simulink model "atrias_HW_boom_nmSt_kinSw_v4"  (R2015a)
settings: Solver=ode4  StartTime=0.0  StopTime=inf  FixedStep=sample_time  RelTol=1e-3
values from neighbouring files (symbols this model uses):
  control_start_time = 15    [setParams.m]
  flag_CtrlMode = 0    [setParams.m]
  kinSw_alpha_start = 130*pi/180    (= 2.26892802759)    [setParams.m]
  kinSw_alpha_tgt = 70*pi/180    (= 1.2217304764)    [setParams.m]
  kinSw_t_start = 0.5    [setParams.m]
  poser_LLegAlp = (initial_l_leg_angle -pi/2)*180/pi    (= 105)    [setParams.m]
  poser_LLegLen = initial_l_leg_length    (= 0.8)    [setParams.m]
  poser_RLegAlp = (initial_r_leg_angle -pi/2)*180/pi    (= 75)    [setParams.m]
  poser_RLegLen = initial_r_leg_length    (= 0.8)    [setParams.m]
  tune_kinSw_alpha_start = kinSw_alpha_start*180/pi    (= 130)    [setParams.m]
  tune_kinSw_alpha_tgt = kinSw_alpha_tgt*180/pi    (= 70)    [setParams.m]
  tune_kinSw_gClr_tgt = kinSw_gClr    (= 0.15)    [setParams.m]
  tune_kinSw_gH_tgt = kinSw_gH_tgt    (= -0.01)    [setParams.m]
  tune_M1_G = 9.5    [setParams.m]
  tune_M3_0 = CtrlPar_theta0*180/pi    [setParams.m]
  tune_M3_D = St_GainDTh_HFL*5    [setParams.m]
  tune_M3_P = St_GainTh_HFL*5    [setParams.m]
  tune_M4_G = 1    [setParams.m]
undefined symbols (not defined in the file or in its folder): A1_notch_f1, A2_notch_f1, A_kalman_fourbar_gear, A_lpf_dtau, B1_lpf_dtau, B1_notch_f1, B2_lpf_dtau, B2_notch_f1, B_kalman_fourbar_gear, boom_mount_angle, boom_mount_to_center_diagonal, c_jointstop, C_kalman_fourbar_gear, contactThr, d_vertical_com, delta_phi_max, delta_phi_max_buffer, delta_phi_max_dropoff, delta_phi_min, Discrete, FmaxBFSH, FmaxGLU, FmaxHAM, FmaxHFL, FmaxRF, FmaxVAS, FPCtrlPar, g, gain_nodes_sea_torque, HIP_MTR_MAX_CONT_TORQUE, initial_dx_estimate, j_motor, k_leg_spring, K_notch_f1, k_sea, kalman_load_to_deflect_transmission, kd_lateral, kd_motor, kd_shin_max, kd_shin_min, kd_splay_max, kd_splay_min, kd_thigh_max, kd_thigh_min, kp_lateral, kp_motor, kp_sea_torque, kp_shin_max, kp_shin_min, kp_splay_max, kp_splay_min, kp_thigh_max, kp_thigh_min, l_boom, l_seg, l_v, lateral_motor_efficiency, lateral_offset, lateral_target_angle_right, lateral_transition_force ... (+123)
libraries: simulink_extras x28, simulink x11, ctrlSharedLib x4
(part 5 of 8)

== system atrias_HW_boom_nmSt_kinSw_v4/Control/Behavior Control/Virtual Neuromuscular Control/Neural Control Layer/L Stance Phase (sagittal) ==
  note: Left Stance Phase Control
  note: 0: Prestimulations
  note: M1: realize compliant leg
  note: M2: prevent knee overextension
  note: M3: balance trunk
  CtrlPar : Inport
  theta_tgt [rad] : Inport  Port=2
  theta dtheta [rad rad/s] : Inport  Port=3
  FmVAS : Inport  Port=4
  LceBFSH : Inport  Port=5
  Enable : EnablePort  StatesWhenEnabling=reset  ZeroCross=off
  Demux2 : Demux
  Demux5 : Demux  Outputs=5
  Demux7 : Demux  Outputs=2
  Divide{4..6,8,13,15,19..20} (8 alike) : Product
  Gain : Gain  Gain=-1
  Gain2 : Gain  Gain=-1
  Gain3 : Gain  Gain=-1
  Mux1 : Mux  Inputs=3
  Mux2 : Mux  Inputs=2
  Sum1 : Sum  Inputs=-+|  SaturateOnIntegerOverflow=on  InputSameDT=on  OutDataTypeStr=Inherit: Same as first input
  Sum2 : Sum  Inputs=|++  SaturateOnIntegerOverflow=on  InputSameDT=on  OutDataTypeStr=Inherit: Same as first input
  Sum3 : Sum  Inputs=-+|  SaturateOnIntegerOverflow=on  InputSameDT=on  OutDataTypeStr=Inherit: Same as first input
  Sum4 : Sum  Inputs=-+|  SaturateOnIntegerOverflow=on  InputSameDT=on  OutDataTypeStr=Inherit: Same as first input
  Sum8 : Sum  Inputs=|++  SaturateOnIntegerOverflow=on  InputSameDT=on  OutDataTypeStr=Inherit: Same as first input
  parStPreS : Selector  InputPortWidth=St_i  Indices=parSt_PreS_i
  parSt_M1 : Selector  InputPortWidth=St_i  Indices=parSt_M1_i
  parSt_M2 : Selector  InputPortWidth=St_i  Indices=parSt_M2_i
  parSt_M3 : Selector  InputPortWidth=St_i  Indices=parSt_M3_i
  positive half{1..4,6} (5 alike) : Saturate  UpperLimit=inf  LowerLimit=0  ZeroCross=off
  S_St_0 : Outport  OutputWhenDisabled=reset  InitialOutput=0
  S_M1 [VAS] : Outport  Port=2  OutputWhenDisabled=reset  InitialOutput=0
  S_M2 [VAS BFSH] : Outport  Port=3  OutputWhenDisabled=reset  InitialOutput=0
  S_M3 [HFL GLU HAM] : Outport  Port=4  OutputWhenDisabled=reset  InitialOutput=0
  wires:
  CtrlPar/1 -> parStPreS/1, parSt_M3/1, parSt_M2/1, parSt_M1/1
  parStPreS/1 -> S_St_0/1
  parSt_M1/1 -> Divide8/1  "FGain_VAS"
  Divide8/1 -> S_M1 [VAS]/1  "VAS"
  FmVAS/1 -> Divide8/2
  parSt_M2/1 -> Demux2/1
  Sum3/1 -> positive half3/1
  Demux2/2 -> Divide15/2  "LGainBFSH_VAS"
  Demux2/4 -> Divide13/2  "LGain_BFSH"
  positive half3/1 -> Divide15/1
  Demux2/1 -> Sum3/1  "loff_BFSH_VAS"
  Divide15/1 -> Gain/1
  Divide13/1 -> Mux2/2  "BFSH"
  Gain/1 -> Mux2/1  "VAS"
  Sum4/1 -> positive half4/1
  positive half4/1 -> Divide13/1
  Demux2/3 -> Sum4/1  "loff_BFSH"
  LceBFSH/1 -> Sum3/2, Sum4/2
  Mux2/1 -> S_M2 [VAS BFSH]/1
  parSt_M3/1 -> Demux5/1
  Demux5/1 -> Divide19/2  "GainTh_HFL"
  Demux5/2 -> Divide20/2  "GainDTh_HFL"
  Demux5/3 -> Divide4/2  "GainTh_GLU"
  Demux5/4 -> Divide5/2  "GainDTh_GLU"
  theta dtheta [rad rad/s]/1 -> Demux7/1
  Demux7/1 -> Sum1/2  "theta"
  Demux7/2 -> Gain3/1, Divide5/1  "dtheta"
  Sum1/1 -> Gain2/1, Divide4/1
  Gain2/1 -> Divide19/1
  Gain3/1 -> Divide20/1
  Divide19/1 -> Sum2/1
  Divide20/1 -> Sum2/2
  Divide4/1 -> Sum8/1
  Divide5/1 -> Sum8/2
  Sum2/1 -> positive half1/1  "HFL"
  Sum8/1 -> Divide6/1, positive half2/1  "GLU"
  Mux1/1 -> S_M3 [HFL GLU HAM]/1
  Demux5/5 -> Divide6/2  "SGainGLU_HAM"
  Divide6/1 -> positive half6/1  "HAM"
  theta_tgt [rad]/1 -> Sum1/1
  positive half1/1 -> Mux1/1
  positive half2/1 -> Mux1/2
  positive half6/1 -> Mux1/3

== system atrias_HW_boom_nmSt_kinSw_v4/Control/Behavior Control/Virtual Neuromuscular Control/Neural Control Layer/L Stance, Swing, Trans (sagittal) ==
  note: Stance DS1 Swing DS2
  note: FullStance Swing
  note: |------------------------------|--------------------|
  note: |--------------------|------------------------------|
  ILLoad : Inport
  S_0_St : Inport  Port=2
  S_M1 : Inport  Port=3
  S_M2 : Inport  Port=4
  S_M3 : Inport  Port=5
  Add3 : Sum  Inputs=2
  Demux2 : Demux  Outputs=2
  Demux3 : Demux  Outputs=3
  Divide17 : Product
  Mux1 : Mux  Inputs=7
  Mux6 : Mux  Inputs=6
  RF : Constant  Value=0
  Sum6 : Sum  Inputs=++|  SaturateOnIntegerOverflow=on  InputSameDT=on  OutDataTypeStr=Inherit: Same as first input
  S : Outport  OutputWhenDisabled=reset  InitialOutput=0
  S_Modules : Outport  Port=2  OutputWhenDisabled=reset  InitialOutput=0
  wires:
  [M3_HFL] -> Mux6/1  "HFL"
  [M3_GLU] -> Mux6/2  "GLU"
  [M3_HAM] -> Mux6/3  "HAM"
  Add3/1 -> Mux6/5  "VAS"
  [M2_BFSH] -> Mux6/6  "KFL"
  Mux6/1 -> Sum6/2
  Sum6/1 -> S/1
  S_0_St/1 -> Sum6/1, [M0_St]
  S_M1/1 -> [M1_VAS]  "VAS"
  S_M2/1 -> Demux2/1  "VAS BFSH"
  Demux2/1 -> [M2_VAS]  "M2_VAS"
  Demux2/2 -> [M2_BFSH]  "M2_BFSH"
  S_M3/1 -> Divide17/1
  ILLoad/1 -> Divide17/2
  Divide17/1 -> Demux3/1
  Demux3/1 -> [M3_HFL]  "M3_HFL"
  Demux3/2 -> [M3_GLU]  "M3_GLU"
  Demux3/3 -> [M3_HAM]  "M3_HAM"
  [M1_VAS] -> Add3/1
  [M2_VAS] -> Add3/2
  [M3_HFL] -> Mux1/5  "10"
  [M3_GLU] -> Mux1/6  "11"
  [M3_HAM] -> Mux1/7  "12"
  [M2_VAS] -> Mux1/3  "8"
  [M2_BFSH] -> Mux1/4  "9"
  [M1_VAS] -> Mux1/2  "7"
  [M0_St] -> Mux1/1  "1~6"
  Mux1/1 -> S_Modules/1
  RF/1 -> Mux6/4

== system atrias_HW_boom_nmSt_kinSw_v4/Control/Behavior Control/Virtual Neuromuscular Control/Neural Control Layer/R Stance Phase (sagittal) ==
  note: Left Stance Phase Control
  note: 0: Prestimulations
  note: M1: realize compliant leg
  note: M2: prevent knee overextension
  note: M3: balance trunk
  CtrlPar : Inport
  theta_tgt [rad] : Inport  Port=2
  theta dtheta [rad rad/s] : Inport  Port=3
  FmVAS : Inport  Port=4
  LceBFSH : Inport  Port=5
  Enable : EnablePort  StatesWhenEnabling=reset  ZeroCross=off
  Demux2 : Demux
  Demux5 : Demux  Outputs=5
  Demux7 : Demux  Outputs=2
  Divide{4..6,8,13,15,19..20} (8 alike) : Product
  Gain : Gain  Gain=-1
  Gain2 : Gain  Gain=-1
  Gain3 : Gain  Gain=-1
  Mux1 : Mux  Inputs=3
  Mux2 : Mux  Inputs=2
  Sum1 : Sum  Inputs=-+|  SaturateOnIntegerOverflow=on  InputSameDT=on  OutDataTypeStr=Inherit: Same as first input
  Sum2 : Sum  Inputs=|++  SaturateOnIntegerOverflow=on  InputSameDT=on  OutDataTypeStr=Inherit: Same as first input
  Sum3 : Sum  Inputs=-+|  SaturateOnIntegerOverflow=on  InputSameDT=on  OutDataTypeStr=Inherit: Same as first input
  Sum4 : Sum  Inputs=-+|  SaturateOnIntegerOverflow=on  InputSameDT=on  OutDataTypeStr=Inherit: Same as first input
  Sum8 : Sum  Inputs=|++  SaturateOnIntegerOverflow=on  InputSameDT=on  OutDataTypeStr=Inherit: Same as first input
  parStPreS : Selector  InputPortWidth=St_i  Indices=parSt_PreS_i
  parSt_M1 : Selector  InputPortWidth=St_i  Indices=parSt_M1_i
  parSt_M2 : Selector  InputPortWidth=St_i  Indices=parSt_M2_i
  parSt_M3 : Selector  InputPortWidth=St_i  Indices=parSt_M3_i
  positive half{1..4,6} (5 alike) : Saturate  UpperLimit=inf  LowerLimit=0  ZeroCross=off
  S_St_0 : Outport  OutputWhenDisabled=reset  InitialOutput=0
  S_M1 [VAS] : Outport  Port=2  OutputWhenDisabled=reset  InitialOutput=0
  S_M2 [VAS BFSH] : Outport  Port=3  OutputWhenDisabled=reset  InitialOutput=0
  S_M3 [HFL GLU HAM] : Outport  Port=4  OutputWhenDisabled=reset  InitialOutput=0
  wires:
  CtrlPar/1 -> parStPreS/1, parSt_M3/1, parSt_M2/1, parSt_M1/1
  parStPreS/1 -> S_St_0/1
  parSt_M1/1 -> Divide8/1  "FGain_VAS"
  Divide8/1 -> S_M1 [VAS]/1  "VAS"
  FmVAS/1 -> Divide8/2
  parSt_M2/1 -> Demux2/1
  Sum3/1 -> positive half3/1
  Demux2/2 -> Divide15/2  "LGainBFSH_VAS"
  Demux2/4 -> Divide13/2  "LGain_BFSH"
  positive half3/1 -> Divide15/1
  Demux2/1 -> Sum3/1  "loff_BFSH_VAS"
  Divide15/1 -> Gain/1
  Divide13/1 -> Mux2/2  "BFSH"
  Gain/1 -> Mux2/1  "VAS"
  Sum4/1 -> positive half4/1
  positive half4/1 -> Divide13/1
  Demux2/3 -> Sum4/1  "loff_BFSH"
  LceBFSH/1 -> Sum3/2, Sum4/2
  Mux2/1 -> S_M2 [VAS BFSH]/1
  parSt_M3/1 -> Demux5/1
  Demux5/1 -> Divide19/2  "GainTh_HFL"
  Demux5/2 -> Divide20/2  "GainDTh_HFL"
  Demux5/3 -> Divide4/2  "GainTh_GLU"
  Demux5/4 -> Divide5/2  "GainDTh_GLU"
  theta dtheta [rad rad/s]/1 -> Demux7/1
  Demux7/1 -> Sum1/2  "theta"
  Demux7/2 -> Gain3/1, Divide5/1  "dtheta"
  Sum1/1 -> Gain2/1, Divide4/1
  Gain2/1 -> Divide19/1
  Gain3/1 -> Divide20/1
  Divide19/1 -> Sum2/1
  Divide20/1 -> Sum2/2
  Divide4/1 -> Sum8/1
  Divide5/1 -> Sum8/2
  Sum2/1 -> positive half1/1  "HFL"
  Sum8/1 -> Divide6/1, positive half2/1  "GLU"
  Mux1/1 -> S_M3 [HFL GLU HAM]/1
  Demux5/5 -> Divide6/2  "SGainGLU_HAM"
  Divide6/1 -> positive half6/1  "HAM"
  theta_tgt [rad]/1 -> Sum1/1
  positive half1/1 -> Mux1/1
  positive half2/1 -> Mux1/2
  positive half6/1 -> Mux1/3

== system atrias_HW_boom_nmSt_kinSw_v4/Control/Behavior Control/Virtual Neuromuscular Control/Neural Control Layer/R Stance, Swing, Trans (sagittal) ==
  note: Stance DS1 Swing DS2
  note: FullStance Swing
  note: |------------------------------|--------------------|
  note: |--------------------|------------------------------|
  ILLoad : Inport
  S_0_St : Inport  Port=2
  S_M1 : Inport  Port=3
  S_M2 : Inport  Port=4
  S_M3 : Inport  Port=5
  Add3 : Sum  Inputs=2
  Demux2 : Demux  Outputs=2
  Demux3 : Demux  Outputs=3
  Divide17 : Product
  Mux1 : Mux  Inputs=7
  Mux6 : Mux  Inputs=6
  RF : Constant  Value=0
  Sum6 : Sum  Inputs=++|  SaturateOnIntegerOverflow=on  InputSameDT=on  OutDataTypeStr=Inherit: Same as first input
  S : Outport  OutputWhenDisabled=reset  InitialOutput=0
  S_Modules : Outport  Port=2  OutputWhenDisabled=reset  InitialOutput=0
  wires:
  [M3_HFL] -> Mux6/1  "HFL"
  [M3_GLU] -> Mux6/2  "GLU"
  [M3_HAM] -> Mux6/3  "HAM"
  Add3/1 -> Mux6/5  "VAS"
  [M2_BFSH] -> Mux6/6  "KFL"
  Mux6/1 -> Sum6/2
  Sum6/1 -> S/1
  S_0_St/1 -> Sum6/1, [M0_St]
  S_M1/1 -> [M1_VAS]  "VAS"
  S_M2/1 -> Demux2/1  "VAS BFSH"
  Demux2/1 -> [M2_VAS]  "M2_VAS"
  Demux2/2 -> [M2_BFSH]  "M2_BFSH"
  S_M3/1 -> Divide17/1
  ILLoad/1 -> Divide17/2
  Divide17/1 -> Demux3/1
  Demux3/1 -> [M3_HFL]  "M3_HFL"
  Demux3/2 -> [M3_GLU]  "M3_GLU"
  Demux3/3 -> [M3_HAM]  "M3_HAM"
  [M1_VAS] -> Add3/1
  [M2_VAS] -> Add3/2
  [M3_HFL] -> Mux1/5  "10"
  [M3_GLU] -> Mux1/6  "11"
  [M3_HAM] -> Mux1/7  "12"
  [M2_VAS] -> Mux1/3  "8"
  [M2_BFSH] -> Mux1/4  "9"
  [M1_VAS] -> Mux1/2  "7"
  [M0_St] -> Mux1/1  "1~6"
  Mux1/1 -> S_Modules/1
  RF/1 -> Mux6/4

== system atrias_HW_boom_nmSt_kinSw_v4/Control/Behavior Control/Virtual Neuromuscular Control/Torque Distribution/mech limit avoidance1 ==
  tau_des [Nm]x4 : Inport
  PD Joint Limit : Subsystem
  PD Joint Limit1 : Subsystem  Commented=on
  Product : Product
  Sum : Sum  Inputs=++|
  tau_des + pd [Nm]x4 : Outport
  wires:
  Product/1 -> Sum/2
  PD Joint Limit/2(des_trq_scale x4) -> Product/1
  Sum/1 -> tau_des + pd [Nm]x4/1
  PD Joint Limit/1(tau_pd_hip_knee [Nm]x4) -> Sum/1
  tau_des [Nm]x4/1 -> Product/2

== system atrias_HW_boom_nmSt_kinSw_v4/Control/Behavior Control/command routing/(M4) Swing Leg Complensation/Swing Leg Compensation ==
  StTorques : Inport
  SwTorques : Inport  Port=2
  M4_G : Inport  Port=3
  Demux : Demux  Outputs=2
  Demux1 : Demux  Outputs=2
  Divide : Product
  Gain : Gain  Gain=.5
  Mux : Mux  Inputs=2
  Sum : Sum  Inputs=|++
  Sum1 : Sum  Inputs=|++
  Sum2 : Sum  Inputs=|++
  StTorques_comp : Outport
  SwTorques_comp : Outport  Port=2
  wires:
  Demux1/1 -> Sum1/1
  Sum/1 -> Gain/1  "SwLegTorque"
  Demux/1 -> Sum/1
  Demux1/2 -> Sum2/1
  Demux/2 -> Sum/2
  StTorques/1 -> Demux1/1
  Mux/1 -> StTorques_comp/1  "StTorques_comp"
  SwTorques/1 -> Demux/1, SwTorques_comp/1
  Sum2/1 -> Mux/2
  Divide/1 -> Sum1/2, Sum2/2
  Sum1/1 -> Mux/1
  Gain/1 -> Divide/1
  M4_G/1 -> Divide/2

== system atrias_HW_boom_nmSt_kinSw_v4/Control/Behavior Control/kinematic swing leg controller/Back//Front Motor PD/Friction Compensation ==
  Right/Left [1/0] : Inport
  Commanded Velocity [rad/s] [back front] : Inport  Port=2
  Product : Product
  Sign : Signum
  Sum1 : Sum
  Switch : Switch  Criteria=u2 ~= 0
  Switch1 : Switch  Criteria=u2 ~= 0
  coulomb_friction_left : Constant  Value=sea_coulomb_friction(3:4)
  coulomb_friction_right : Constant  Value=sea_coulomb_friction(1:2)
  offset_friction_left : Constant  Value=sea_offset_friction(3:4)
  offset_friction_right : Constant  Value=sea_offset_friction(1:2)
  Friction Compensation [Nm] : Outport
  wires:
  Commanded Velocity [rad/s] [back front]/1 -> Sign/1
  Switch/1 -> Sum1/2
  Sum1/1 -> Friction Compensation [Nm]/1
  Product/1 -> Sum1/1
  Right/Left [1/0]/1 -> Switch1/2, Switch/2
  offset_friction_right/1 -> Switch/1
  offset_friction_left/1 -> Switch/3
  coulomb_friction_right/1 -> Switch1/1
  coulomb_friction_left/1 -> Switch1/3
  Switch1/1 -> Product/2
  Sign/1 -> Product/1

== system atrias_HW_boom_nmSt_kinSw_v4/Control/Poser/Subsystem/Back//Front Motor PD/Friction Compensation ==
  Right/Left [1/0] : Inport
  Commanded Velocity [rad/s] [back front] : Inport  Port=2
  Product : Product
  Sign : Signum
  Sum1 : Sum
  Switch : Switch  Criteria=u2 ~= 0
  Switch1 : Switch  Criteria=u2 ~= 0
  coulomb_friction_left : Constant  Value=sea_coulomb_friction(3:4)
  coulomb_friction_right : Constant  Value=sea_coulomb_friction(1:2)
  offset_friction_left : Constant  Value=sea_offset_friction(3:4)
  offset_friction_right : Constant  Value=sea_offset_friction(1:2)
  Friction Compensation [Nm] : Outport
  wires:
  Commanded Velocity [rad/s] [back front]/1 -> Sign/1
  Switch/1 -> Sum1/2
  Sum1/1 -> Friction Compensation [Nm]/1
  Product/1 -> Sum1/1
  Right/Left [1/0]/1 -> Switch1/2, Switch/2
  offset_friction_right/1 -> Switch/1
  offset_friction_left/1 -> Switch/3
  coulomb_friction_right/1 -> Switch1/1
  coulomb_friction_left/1 -> Switch1/3
  Switch1/1 -> Product/2
  Sign/1 -> Product/1

== system atrias_HW_boom_nmSt_kinSw_v4/Control/Poser/Subsystem/Back//Front Motor PD1/Friction Compensation ==
  Right/Left [1/0] : Inport
  Commanded Velocity [rad/s] [back front] : Inport  Port=2
  Product : Product
  Sign : Signum
  Sum1 : Sum
  Switch : Switch  Criteria=u2 ~= 0
  Switch1 : Switch  Criteria=u2 ~= 0
  coulomb_friction_left : Constant  Value=sea_coulomb_friction(3:4)
  coulomb_friction_right : Constant  Value=sea_coulomb_friction(1:2)
  offset_friction_left : Constant  Value=sea_offset_friction(3:4)
  offset_friction_right : Constant  Value=sea_offset_friction(1:2)
  Friction Compensation [Nm] : Outport
  wires:
  Commanded Velocity [rad/s] [back front]/1 -> Sign/1
  Switch/1 -> Sum1/2
  Sum1/1 -> Friction Compensation [Nm]/1
  Product/1 -> Sum1/1
  Right/Left [1/0]/1 -> Switch1/2, Switch/2
  offset_friction_right/1 -> Switch/1
  offset_friction_left/1 -> Switch/3
  coulomb_friction_right/1 -> Switch1/1
  coulomb_friction_left/1 -> Switch1/3
  Switch1/1 -> Product/2
  Sign/1 -> Product/1

== system atrias_HW_boom_nmSt_kinSw_v4/Control/Behavior Control/Add Limit Avoidance PD Torques/mechanical limit avoidance/PD Joint Limit/L Scale desired torque ==
  note: NOTE: min_splay_angle does not equal delta_phi_min
  phi_thigh [rad] : Inport
  phi_shin [rad] : Inport  Port=2
  Constant : Constant
  Constant1 : Constant  Value=delta_phi_max - delta_phi_max_buffer
  Constant10 : Constant  Value=phi_thigh_max_dropoff
  Constant11 : Constant  Value=phi_shin_min_dropoff
  Constant12 : Constant  Value=phi_shin_max_dropoff
  Constant13 : Constant
  Constant2 : Constant  Value=phi_thigh_max - phi_thigh_max_buffer
  Constant3 : Constant  Value=min_splay_angle+min_splay_buffer
  Constant4 : Constant  Value=phi_thigh_min + phi_thigh_min_buffer
  Constant5 : Constant  Value=phi_shin_max - phi_shin_max_buffer
  Constant6 : Constant  Value=phi_shin_min + phi_shin_min_buffer
  Constant7 : Constant  Value=min_splay_dropoff
  Constant8 : Constant  Value=delta_phi_max_dropoff
  Constant9 : Constant  Value=phi_thigh_min_dropoff
  Divide{,1..5} (6 alike) : Product  Inputs=/*
  Gain : Gain  Gain=-1
  Gain1 : Gain  Gain=-1
  Gain2 : Gain  Gain=-1
  L PD scale : Scope  NumInputPorts=4
      settings: ShowLegends=on  TimeRange=2.5  YMin=-100~-5e+07~-1e+07~-5  YMax=100~1e+07~5e+07~5  SaveName=ScopeData5
  Mux{,1,7..8} (4 alike) : Mux  Inputs=2
  Sum : Sum  Inputs=|+-
  Sum1 : Sum  Inputs=-+|
  Sum2 : Sum  Inputs=+-
  Sum{3..8} (6 alike) : Sum  Inputs=+-|
  [0,1]{,1..5} (6 alike) : Saturate  UpperLimit=1  LowerLimit=0
  max : MinMax  Function=max  Inputs=4
  max2 : MinMax  Function=max  Inputs=4
  scale_back : Outport
  scale_front : Outport  Port=2
  wires:
  Mux1/1 -> L PD scale/4
  Sum1/1 -> scale_front/1, Mux1/2
  [min_thigh_scale] -> max2/3
  [max_thigh_scale] -> max2/4
  [max_splay_scale] -> max/4, max2/2
  [min_splay_scale] -> max/3, max2/1
  [max_shin_scale] -> max/2
  [min_shin_scale] -> max/1
  max2/1 -> Sum1/1
  Constant13/1 -> Sum1/2
  Gain2/1 -> Divide5/2
  Constant12/1 -> Divide5/1
  Sum7/1 -> Gain2/1
  "[0,1]5"/1 -> [max_shin_scale]
  Divide5/1 -> "[0,1]5"/1
  Constant11/1 -> Divide4/1
  Sum8/1 -> Divide4/2
  "[0,1]4"/1 -> [min_shin_scale]
  Divide4/1 -> "[0,1]4"/1
  Constant10/1 -> Divide3/1
  Sum5/1 -> Gain1/1
  Gain1/1 -> Divide3/2
  "[0,1]3"/1 -> [max_thigh_scale]
  Divide3/1 -> "[0,1]3"/1
  Constant9/1 -> Divide2/1
  Sum6/1 -> Divide2/2
  "[0,1]2"/1 -> [min_thigh_scale]
  Divide2/1 -> "[0,1]2"/1
  Gain/1 -> Divide1/2
  Constant8/1 -> Divide1/1
  Sum3/1 -> Gain/1
  "[0,1]1"/1 -> [max_splay_scale]
  Divide1/1 -> "[0,1]1"/1
  "[0,1]"/1 -> [min_splay_scale]
  Divide/1 -> "[0,1]"/1
  Sum4/1 -> Divide/2
  Constant7/1 -> Divide/1
  max/1 -> Sum/2
  Constant/1 -> Sum/1
  Sum/1 -> scale_back/1, Mux1/1
  [max_splay_scale] -> Mux7/2  "max_splay_trq"
  [min_splay_scale] -> Mux7/1  "min_splay_trq"
  Mux7/1 -> L PD scale/3
  Mux8/1 -> L PD scale/2
  [max_shin_scale] -> Mux8/2  "max_shin_trq"
  [min_shin_scale] -> Mux8/1  "min_shin_trq"
  Mux/1 -> L PD scale/1
  [max_thigh_scale] -> Mux/2  "max_thigh_trq"
  [min_thigh_scale] -> Mux/1  "min_thigh_trq"
  Constant5/1 -> Sum7/1
  [shin] -> Sum7/2
  Constant6/1 -> Sum8/1
  [shin] -> Sum8/2
  Constant2/1 -> Sum5/1
  [thigh] -> Sum5/2
  Constant4/1 -> Sum6/1
  [thigh] -> Sum6/2
  Constant1/1 -> Sum3/1
  [splay] -> Sum3/2
  Constant3/1 -> Sum4/1
  [splay] -> Sum4/2
  Sum2/1 -> [splay]  "splay angle"
  phi_thigh [rad]/1 -> Sum2/2, [thigh]
  phi_shin [rad]/1 -> Sum2/1, [shin]

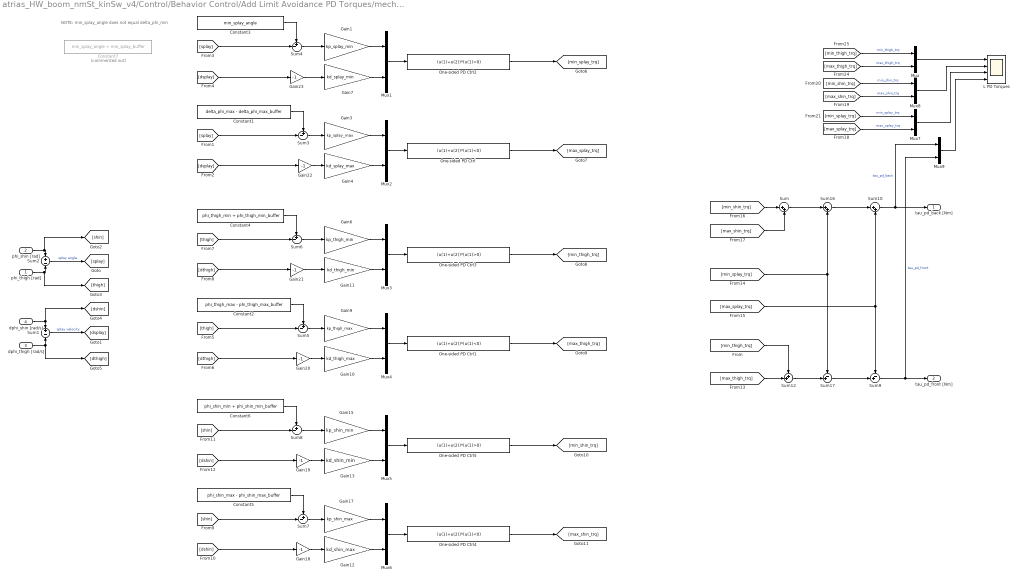
== system atrias_HW_boom_nmSt_kinSw_v4/Control/Behavior Control/Add Limit Avoidance PD Torques/mechanical limit avoidance/PD Joint Limit/L mechanical Limit Avoidance Torques (Virtual) ==
  note: NOTE: min_splay_angle does not equal delta_phi_min
  phi_thigh [rad] : Inport
  phi_shin [rad] : Inport  Port=2
  dphi_thigh [rad/s] : Inport  Port=3
  dphi_shin [rad/s] : Inport  Port=4
  Constant1 : Constant  Value=delta_phi_max - delta_phi_max_buffer
  Constant2 : Constant  Value=phi_thigh_max - phi_thigh_max_buffer
  Constant3 : Constant  Value=min_splay_angle
  Constant4 : Constant  Value=phi_thigh_min + phi_thigh_min_buffer
  Constant5 : Constant  Value=phi_shin_max - phi_shin_max_buffer
  Constant6 : Constant  Value=phi_shin_min + phi_shin_min_buffer
  Constant7 : Constant  Commented=on  Value=min_splay_angle + min_splay_buffer
  Gain1 : Gain  Gain=kp_splay_min
  Gain10 : Gain  Gain=kd_thigh_max
  Gain11 : Gain  Gain=kd_thigh_min
  Gain12 : Gain  Gain=kd_shin_max
  Gain13 : Gain  Gain=kd_shin_min
  Gain15 : Gain  Gain=kp_shin_min
  Gain17 : Gain  Gain=kp_shin_max
  Gain{18..23} (6 alike) : Gain  Gain=-1
  Gain3 : Gain  Gain=kp_splay_max
  Gain4 : Gain  Gain=kd_splay_max
  Gain6 : Gain  Gain=kp_thigh_min
  Gain7 : Gain  Gain=kd_splay_min
  Gain9 : Gain  Gain=kp_thigh_max
  L PD Torques : Scope  NumInputPorts=4
      settings: ShowLegends=on  TimeRange=2.5  YMin=-100~-5e+07~-1e+07~-5  YMax=100~1e+07~5e+07~5  SaveName=ScopeData5
  Mux{,1..9} (10 alike) : Mux  Inputs=2
  One-sided PD Ctrl : Fcn  Expr=(u(1)+u(2))*(u(1)<0)
  One-sided PD Ctrl1 : Fcn  Expr=(u(1)+u(2))*(u(1)<0)
  One-sided PD Ctrl2 : Fcn  Expr=(u(1)+u(2))*(u(1)>0)
  One-sided PD Ctrl3 : Fcn  Expr=(u(1)+u(2))*(u(1)>0)
  One-sided PD Ctrl4 : Fcn  Expr=(u(1)+u(2))*(u(1)<0)
  One-sided PD Ctrl5 : Fcn  Expr=(u(1)+u(2))*(u(1)>0)
  Sum : Sum  Inputs=|++
  Sum1 : Sum  Inputs=+-
  Sum10 : Sum  Inputs=|++
  Sum12 : Sum  Inputs=++|
  Sum16 : Sum  Inputs=|++
  Sum17 : Sum  Inputs=-+|
  Sum2 : Sum  Inputs=+-
  Sum{3..8} (6 alike) : Sum  Inputs=+-|
  Sum9 : Sum  Inputs=-+|
  tau_pd_back [Nm] : Outport
  tau_pd_front [Nm] : Outport  Port=2
  wires:
  Mux9/1 -> L PD Torques/4
  dphi_shin [rad/s]/1 -> [dshin], Sum1/1
  dphi_thigh [rad/s]/1 -> [dthigh], Sum1/2
  phi_shin [rad]/1 -> [shin], Sum2/1
  phi_thigh [rad]/1 -> [thigh], Sum2/2
  Sum2/1 -> [splay]  "splay angle"
  Sum1/1 -> [dsplay]  "splay velocity"
  [dsplay] -> Gain23/1
  [splay] -> Sum4/2
  Gain7/1 -> Mux1/2
  Gain1/1 -> Mux1/1
  Sum4/1 -> Gain1/1
  Constant3/1 -> Sum4/1
  Mux1/1 -> One-sided PD Ctrl2/1
  [dsplay] -> Gain22/1
  [splay] -> Sum3/2
  Gain4/1 -> Mux2/2
  Gain3/1 -> Mux2/1
  Sum3/1 -> Gain3/1
  Constant1/1 -> Sum3/1
  Mux2/1 -> One-sided PD Ctrl/1
  [dthigh] -> Gain21/1
  [thigh] -> Sum6/2
  Gain11/1 -> Mux3/2
  Gain6/1 -> Mux3/1
  Sum6/1 -> Gain6/1
  Constant4/1 -> Sum6/1
  Mux3/1 -> One-sided PD Ctrl3/1
  [dthigh] -> Gain20/1
  [thigh] -> Sum5/2
  Gain10/1 -> Mux4/2
  Gain9/1 -> Mux4/1
  Sum5/1 -> Gain9/1
  Constant2/1 -> Sum5/1
  Mux4/1 -> One-sided PD Ctrl1/1
  [dshin] -> Gain19/1
  [shin] -> Sum8/2
  Gain13/1 -> Mux5/2
  Gain15/1 -> Mux5/1
  Sum8/1 -> Gain15/1
  Constant6/1 -> Sum8/1
  Mux5/1 -> One-sided PD Ctrl5/1
  [dshin] -> Gain18/1
  [shin] -> Sum7/2
  Gain12/1 -> Mux6/2
  Gain17/1 -> Mux6/1
  Sum7/1 -> Gain17/1
  Constant5/1 -> Sum7/1
  Mux6/1 -> One-sided PD Ctrl4/1
  One-sided PD Ctrl2/1 -> [min_splay_trq]
  [min_thigh_trq] -> Mux/1  "min_thigh_trq"
  [max_thigh_trq] -> Mux/2  "max_thigh_trq"
  Mux/1 -> L PD Torques/1
  [min_shin_trq] -> Mux8/1  "min_shin_trq"
  [max_shin_trq] -> Mux8/2  "max_shin_trq"
  Mux8/1 -> L PD Torques/2
  Mux7/1 -> L PD Torques/3
  [min_splay_trq] -> Mux7/1  "min_splay_trq"
  [max_splay_trq] -> Mux7/2  "max_splay_trq"
  Sum10/1 -> tau_pd_back [Nm]/1, Mux9/1  "tau_pd_back"
  Sum9/1 -> tau_pd_front [Nm]/1, Mux9/2  "tau_pd_front"
  Sum/1 -> Sum16/1
  [min_shin_trq] -> Sum/1
  [max_shin_trq] -> Sum/2
  Sum16/1 -> Sum10/1
  [min_splay_trq] -> Sum17/1, Sum16/2
  [max_splay_trq] -> Sum9/1, Sum10/2
  [max_thigh_trq] -> Sum12/2
  [min_thigh_trq] -> Sum12/1
  Sum12/1 -> Sum17/2
  Sum17/1 -> Sum9/2
  Gain18/1 -> Gain12/1
  Gain19/1 -> Gain13/1
  Gain20/1 -> Gain10/1
  Gain21/1 -> Gain11/1
  Gain22/1 -> Gain4/1
  Gain23/1 -> Gain7/1
  One-sided PD Ctrl/1 -> [max_splay_trq]
  One-sided PD Ctrl3/1 -> [min_thigh_trq]
  One-sided PD Ctrl1/1 -> [max_thigh_trq]
  One-sided PD Ctrl5/1 -> [min_shin_trq]
  One-sided PD Ctrl4/1 -> [max_shin_trq]

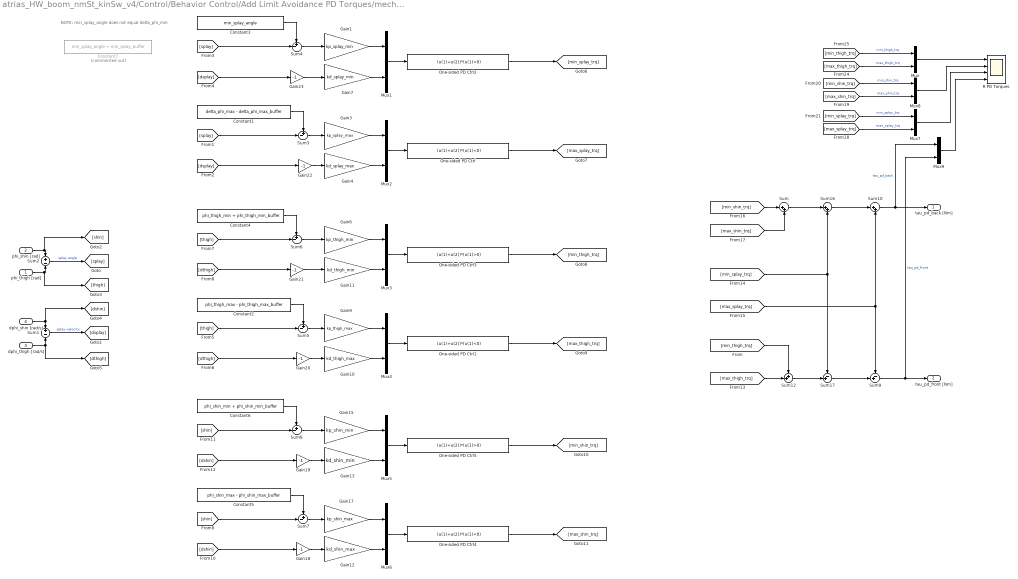
== system atrias_HW_boom_nmSt_kinSw_v4/Control/Behavior Control/Add Limit Avoidance PD Torques/mechanical limit avoidance/PD Joint Limit/R Mechanical Limit Avoidance Torques (Virtual)1 ==
  note: NOTE: min_splay_angle does not equal delta_phi_min
  phi_thigh [rad] : Inport
  phi_shin [rad] : Inport  Port=2
  dphi_thigh [rad/s] : Inport  Port=3
  dphi_shin [rad/s] : Inport  Port=4
  Constant1 : Constant  Value=delta_phi_max - delta_phi_max_buffer
  Constant2 : Constant  Value=phi_thigh_max - phi_thigh_max_buffer
  Constant3 : Constant  Value=min_splay_angle
  Constant4 : Constant  Value=phi_thigh_min + phi_thigh_min_buffer
  Constant5 : Constant  Value=phi_shin_max - phi_shin_max_buffer
  Constant6 : Constant  Value=phi_shin_min + phi_shin_min_buffer
  Constant7 : Constant  Commented=on  Value=min_splay_angle + min_splay_buffer
  Gain1 : Gain  Gain=kp_splay_min
  Gain10 : Gain  Gain=kd_thigh_max
  Gain11 : Gain  Gain=kd_thigh_min
  Gain12 : Gain  Gain=kd_shin_max
  Gain13 : Gain  Gain=kd_shin_min
  Gain15 : Gain  Gain=kp_shin_min
  Gain17 : Gain  Gain=kp_shin_max
  Gain{18..23} (6 alike) : Gain  Gain=-1
  Gain3 : Gain  Gain=kp_splay_max
  Gain4 : Gain  Gain=kd_splay_max
  Gain6 : Gain  Gain=kp_thigh_min
  Gain7 : Gain  Gain=kd_splay_min
  Gain9 : Gain  Gain=kp_thigh_max
  Mux{,1..9} (10 alike) : Mux  Inputs=2
  One-sided PD Ctrl : Fcn  Expr=(u(1)+u(2))*(u(1)<0)
  One-sided PD Ctrl1 : Fcn  Expr=(u(1)+u(2))*(u(1)<0)
  One-sided PD Ctrl2 : Fcn  Expr=(u(1)+u(2))*(u(1)>0)
  One-sided PD Ctrl3 : Fcn  Expr=(u(1)+u(2))*(u(1)>0)
  One-sided PD Ctrl4 : Fcn  Expr=(u(1)+u(2))*(u(1)<0)
  One-sided PD Ctrl5 : Fcn  Expr=(u(1)+u(2))*(u(1)>0)
  R PD Torques : Scope  NumInputPorts=4
      settings: ShowLegends=on  TimeRange=2.5  YMin=-100~-5e+07~-1e+07~-5  YMax=100~1e+07~5e+07~5  SaveName=ScopeData5
  Sum : Sum  Inputs=|++
  Sum1 : Sum  Inputs=+-
  Sum10 : Sum  Inputs=|++
  Sum12 : Sum  Inputs=++|
  Sum16 : Sum  Inputs=|++
  Sum17 : Sum  Inputs=-+|
  Sum2 : Sum  Inputs=+-
  Sum{3..8} (6 alike) : Sum  Inputs=+-|
  Sum9 : Sum  Inputs=-+|
  tau_pd_back [Nm] : Outport
  tau_pd_front [Nm] : Outport  Port=2
  wires:
  One-sided PD Ctrl4/1 -> [max_shin_trq]
  One-sided PD Ctrl5/1 -> [min_shin_trq]
  One-sided PD Ctrl1/1 -> [max_thigh_trq]
  One-sided PD Ctrl3/1 -> [min_thigh_trq]
  One-sided PD Ctrl/1 -> [max_splay_trq]
  Gain23/1 -> Gain7/1
  Gain22/1 -> Gain4/1
  Gain21/1 -> Gain11/1
  Gain20/1 -> Gain10/1
  Gain19/1 -> Gain13/1
  Gain18/1 -> Gain12/1
  Sum17/1 -> Sum9/2
  Sum12/1 -> Sum17/2
  [min_thigh_trq] -> Sum12/1
  [max_thigh_trq] -> Sum12/2
  [max_splay_trq] -> Sum10/2, Sum9/1
  [min_splay_trq] -> Sum16/2, Sum17/1
  Sum16/1 -> Sum10/1
  [max_shin_trq] -> Sum/2
  [min_shin_trq] -> Sum/1
  Sum/1 -> Sum16/1
  Sum9/1 -> Mux9/2, tau_pd_front [Nm]/1  "tau_pd_front"
  Sum10/1 -> Mux9/1, tau_pd_back [Nm]/1  "tau_pd_back"
  [max_splay_trq] -> Mux7/2  "max_splay_trq"
  [min_splay_trq] -> Mux7/1  "min_splay_trq"
  Mux7/1 -> R PD Torques/3
  Mux8/1 -> R PD Torques/2
  [max_shin_trq] -> Mux8/2  "max_shin_trq"
  [min_shin_trq] -> Mux8/1  "min_shin_trq"
  Mux/1 -> R PD Torques/1
  [max_thigh_trq] -> Mux/2  "max_thigh_trq"
  [min_thigh_trq] -> Mux/1  "min_thigh_trq"
  One-sided PD Ctrl2/1 -> [min_splay_trq]
  Mux6/1 -> One-sided PD Ctrl4/1
  Constant5/1 -> Sum7/1
  Sum7/1 -> Gain17/1
  Gain17/1 -> Mux6/1
  Gain12/1 -> Mux6/2
  [shin] -> Sum7/2
  [dshin] -> Gain18/1
  Mux5/1 -> One-sided PD Ctrl5/1
  Constant6/1 -> Sum8/1
  Sum8/1 -> Gain15/1
  Gain15/1 -> Mux5/1
  Gain13/1 -> Mux5/2
  [shin] -> Sum8/2
  [dshin] -> Gain19/1
  Mux4/1 -> One-sided PD Ctrl1/1
  Constant2/1 -> Sum5/1
  Sum5/1 -> Gain9/1
  Gain9/1 -> Mux4/1
  Gain10/1 -> Mux4/2
  [thigh] -> Sum5/2
  [dthigh] -> Gain20/1
  Mux3/1 -> One-sided PD Ctrl3/1
  Constant4/1 -> Sum6/1
  Sum6/1 -> Gain6/1
  Gain6/1 -> Mux3/1
  Gain11/1 -> Mux3/2
  [thigh] -> Sum6/2
  [dthigh] -> Gain21/1
  Mux2/1 -> One-sided PD Ctrl/1
  Constant1/1 -> Sum3/1
  Sum3/1 -> Gain3/1
  Gain3/1 -> Mux2/1
  Gain4/1 -> Mux2/2
  [splay] -> Sum3/2
  [dsplay] -> Gain22/1
  Mux1/1 -> One-sided PD Ctrl2/1
  Constant3/1 -> Sum4/1
  Sum4/1 -> Gain1/1
  Gain1/1 -> Mux1/1
  Gain7/1 -> Mux1/2
  [splay] -> Sum4/2
  [dsplay] -> Gain23/1
  Sum1/1 -> [dsplay]  "splay velocity"
  Sum2/1 -> [splay]  "splay angle"
  phi_thigh [rad]/1 -> Sum2/2, [thigh]
  phi_shin [rad]/1 -> Sum2/1, [shin]
  dphi_thigh [rad/s]/1 -> Sum1/2, [dthigh]
  dphi_shin [rad/s]/1 -> Sum1/1, [dshin]
  Mux9/1 -> R PD Torques/4

== system atrias_HW_boom_nmSt_kinSw_v4/Control/Behavior Control/Add Limit Avoidance PD Torques/mechanical limit avoidance/PD Joint Limit/R Scale desired torque ==
  note: NOTE: min_splay_angle does not equal delta_phi_min
  phi_thigh [rad] : Inport
  phi_shin [rad] : Inport  Port=2
  Constant : Constant
  Constant1 : Constant  Value=delta_phi_max - delta_phi_max_buffer
  Constant10 : Constant  Value=phi_thigh_max_dropoff
  Constant11 : Constant  Value=phi_shin_min_dropoff
  Constant12 : Constant  Value=phi_shin_max_dropoff
  Constant13 : Constant
  Constant2 : Constant  Value=phi_thigh_max - phi_thigh_max_buffer
  Constant3 : Constant  Value=min_splay_angle+min_splay_buffer
  Constant4 : Constant  Value=phi_thigh_min + phi_thigh_min_buffer
  Constant5 : Constant  Value=phi_shin_max - phi_shin_max_buffer
  Constant6 : Constant  Value=phi_shin_min + phi_shin_min_buffer
  Constant7 : Constant  Value=min_splay_dropoff
  Constant8 : Constant  Value=delta_phi_max_dropoff
  Constant9 : Constant  Value=phi_thigh_min_dropoff
  Divide{,1..5} (6 alike) : Product  Inputs=/*
  Gain : Gain  Gain=-1
  Gain1 : Gain  Gain=-1
  Gain2 : Gain  Gain=-1
  Mux{,1,7..8} (4 alike) : Mux  Inputs=2
  R PD scale : Scope  NumInputPorts=4
      settings: ShowLegends=on  TimeRange=2.5  YMin=-100~-5e+07~-1e+07~-5  YMax=100~1e+07~5e+07~5  SaveName=ScopeData5
  Sum : Sum  Inputs=|+-
  Sum1 : Sum  Inputs=-+|
  Sum2 : Sum  Inputs=+-
  Sum{3..8} (6 alike) : Sum  Inputs=+-|
  [0,1]{,1..5} (6 alike) : Saturate  UpperLimit=1  LowerLimit=0
  max : MinMax  Function=max  Inputs=4
  max2 : MinMax  Function=max  Inputs=4
  scale_back : Outport
  scale_front : Outport  Port=2
  wires:
  phi_shin [rad]/1 -> [shin], Sum2/1
  phi_thigh [rad]/1 -> [thigh], Sum2/2
  Sum2/1 -> [splay]  "splay angle"
  [splay] -> Sum4/2
  Constant3/1 -> Sum4/1
  [splay] -> Sum3/2
  Constant1/1 -> Sum3/1
  [thigh] -> Sum6/2
  Constant4/1 -> Sum6/1
  [thigh] -> Sum5/2
  Constant2/1 -> Sum5/1
  [shin] -> Sum8/2
  Constant6/1 -> Sum8/1
  [shin] -> Sum7/2
  Constant5/1 -> Sum7/1
  [min_thigh_scale] -> Mux/1  "min_thigh_trq"
  [max_thigh_scale] -> Mux/2  "max_thigh_trq"
  Mux/1 -> R PD scale/1
  [min_shin_scale] -> Mux8/1  "min_shin_trq"
  [max_shin_scale] -> Mux8/2  "max_shin_trq"
  Mux8/1 -> R PD scale/2
  Mux7/1 -> R PD scale/3
  [min_splay_scale] -> Mux7/1  "min_splay_trq"
  [max_splay_scale] -> Mux7/2  "max_splay_trq"
  Sum/1 -> Mux1/1, scale_back/1
  Constant/1 -> Sum/1
  max/1 -> Sum/2
  Constant7/1 -> Divide/1
  Sum4/1 -> Divide/2
  Divide/1 -> "[0,1]"/1
  "[0,1]"/1 -> [min_splay_scale]
  Divide1/1 -> "[0,1]1"/1
  "[0,1]1"/1 -> [max_splay_scale]
  Sum3/1 -> Gain/1
  Constant8/1 -> Divide1/1
  Gain/1 -> Divide1/2
  Divide2/1 -> "[0,1]2"/1
  "[0,1]2"/1 -> [min_thigh_scale]
  Sum6/1 -> Divide2/2
  Constant9/1 -> Divide2/1
  Divide3/1 -> "[0,1]3"/1
  "[0,1]3"/1 -> [max_thigh_scale]
  Gain1/1 -> Divide3/2
  Sum5/1 -> Gain1/1
  Constant10/1 -> Divide3/1
  Divide4/1 -> "[0,1]4"/1
  "[0,1]4"/1 -> [min_shin_scale]
  Sum8/1 -> Divide4/2
  Constant11/1 -> Divide4/1
  Divide5/1 -> "[0,1]5"/1
  "[0,1]5"/1 -> [max_shin_scale]
  Sum7/1 -> Gain2/1
  Constant12/1 -> Divide5/1
  Gain2/1 -> Divide5/2
  Constant13/1 -> Sum1/2
  max2/1 -> Sum1/1
  [min_shin_scale] -> max/1
  [max_shin_scale] -> max/2
  [min_splay_scale] -> max2/1, max/3
  [max_splay_scale] -> max2/2, max/4
  [max_thigh_scale] -> max2/4
  [min_thigh_scale] -> max2/3
  Sum1/1 -> Mux1/2, scale_front/1
  Mux1/1 -> R PD scale/4

== system atrias_HW_boom_nmSt_kinSw_v4/Control/Behavior Control/Virtual Neuromuscular Control/Muscle Layer/BFSH/BE force-length relation ==
  note: Buffer Elasticity BE
  lce [lopt] : Inport
  Constant1 : Constant  Value=1-mtu_w
  Math Function : Math  Operator=square  SaturateOnIntegerOverflow=on
  Mux1 : Mux  Inputs=2
  Sum4 : Sum  Inputs=|+-  SaturateOnIntegerOverflow=on  InputSameDT=on  OutDataTypeStr=Inherit: Same as first input
  force above slack length : Fcn  Expr=u(2)*(u(1)<0)
  reference strain [lslack] : Constant  Value=mtu_w/2
  relative strain : Product  Inputs=*/
  fbe [Fmax] : Outport
  wires:
  lce [lopt]/1 -> Sum4/1
  Mux1/1 -> force above slack length/1
  force above slack length/1 -> fbe [Fmax]/1
  Math Function/1 -> Mux1/2
  relative strain/1 -> Math Function/1
  reference strain [lslack]/1 -> relative strain/2
  Sum4/1 -> relative strain/1, Mux1/1
  Constant1/1 -> Sum4/2

== system atrias_HW_boom_nmSt_kinSw_v4/Control/Behavior Control/Virtual Neuromuscular Control/Muscle Layer/BFSH/CE force-length relation ==
  note: CE Force-Length Relationship
  lce [lopt] : Inport
  Abs : Abs
  Constant1 : Constant
  Constant2 : Constant  Value=3
  Gain : Gain  Gain=log(mtu_c)
  Math Function : Math  SaturateOnIntegerOverflow=on
  Math Function1 : Math  Operator=pow  SaturateOnIntegerOverflow=on
  Sum4 : Sum  Inputs=|+-  SaturateOnIntegerOverflow=on  InputSameDT=on  OutDataTypeStr=Inherit: Same as first input
  normalized position : Product  Inputs=*/
  relative width : Constant  Value=mtu_w
  fce [Fmax] : Outport
  wires:
  lce [lopt]/1 -> Sum4/1
  relative width/1 -> normalized position/2
  Constant1/1 -> Sum4/2
  Sum4/1 -> Abs/1
  Abs/1 -> normalized position/1
  normalized position/1 -> Math Function1/1
  Constant2/1 -> Math Function1/2
  Math Function1/1 -> Gain/1
  Gain/1 -> Math Function/1
  Math Function/1 -> fce [Fmax]/1

== system atrias_HW_boom_nmSt_kinSw_v4/Control/Behavior Control/Virtual Neuromuscular Control/Muscle Layer/BFSH/CE inverse force-velocity relation ==
  note: CE Inverse Force-Velocity Relationship
  Fv[Fmax] : Inport
  1 : Product  Inputs=/*
  Constant{1,3..4,8} (4 alike) : Constant
  Constant2 : Constant  Value=mtu_N
  Constant5 : Constant  Value=mtu_N
  Curvature : Gain  Gain=mtu_K  SaturateOnIntegerOverflow=on  OutDataTypeStr=Inherit: Same as input  ParamDataTypeStr=Inherit: Same as input
  Curvature1 : Gain  Gain=7.56*mtu_K  SaturateOnIntegerOverflow=on  OutDataTypeStr=Inherit: Same as input  ParamDataTypeStr=Inherit: Same as input
  Mux : Mux  Inputs=2
  Mux1 : Mux  Inputs=3
  Mux2 : Mux  Inputs=3
  Slope : Gain  Gain=1e-2  SaturateOnIntegerOverflow=on  OutDataTypeStr=Inherit: Same as input  ParamDataTypeStr=Inherit: Same as input
  Sum1 : Sum  Inputs=|++  SaturateOnIntegerOverflow=on  InputSameDT=on  OutDataTypeStr=Inherit: Same as first input
  Sum2 : Sum  SaturateOnIntegerOverflow=on  InputSameDT=on  OutDataTypeStr=Inherit: Same as first input
  Sum3 : Sum  Inputs=++|  SaturateOnIntegerOverflow=on  InputSameDT=on  OutDataTypeStr=Inherit: Same as first input
  Sum4 : Sum  Inputs=|+-  SaturateOnIntegerOverflow=on  InputSameDT=on  OutDataTypeStr=Inherit: Same as first input
  Sum5 : Sum  Inputs=|-+  SaturateOnIntegerOverflow=on  InputSameDT=on  OutDataTypeStr=Inherit: Same as first input
  Sum6 : Sum  Inputs=-+|  SaturateOnIntegerOverflow=on  InputSameDT=on  OutDataTypeStr=Inherit: Same as first input
  Sum7 : Sum  Inputs=|++  SaturateOnIntegerOverflow=on  InputSameDT=on  OutDataTypeStr=Inherit: Same as first input
  Sum8 : Sum  Inputs=+-|  SaturateOnIntegerOverflow=on  InputSameDT=on  OutDataTypeStr=Inherit: Same as first input
  Sum9 : Sum  SaturateOnIntegerOverflow=on  InputSameDT=on  OutDataTypeStr=Inherit: Same as first input
  concentric branch : Fcn  Expr=u(1) * (u(2)<=1)
  excentric branch : Fcn  Expr=u(2) * (u(1)>1)*(u(1)<=u(3))
  excentric overshoot : Fcn  Expr=u(3) * (u(2)>u(1))
  v_concentric : Product  Inputs=*/
  v_excentric <N : Product  Inputs=*/
  v[vmax] : Outport
  wires:
  Curvature/1 -> Sum3/2
  Constant1/1 -> Sum4/2, Sum3/1
  Sum4/1 -> v_concentric/1
  Sum3/1 -> v_concentric/2
  1/1 -> Sum7/1, Curvature1/1
  Constant4/1 -> Sum7/2, Sum8/1
  Curvature1/1 -> Sum8/2
  Sum8/1 -> v_excentric <N/2
  Sum7/1 -> v_excentric <N/1
  v_concentric/1 -> Mux/1
  Fv[Fmax]/1 -> Sum4/1, Curvature/1, Sum6/2, Mux/2, Mux1/1, Mux2/2
  Sum9/1 -> v[vmax]/1
  Sum2/1 -> Sum9/2
  excentric overshoot/1 -> Sum2/2
  Slope/1 -> Sum1/1
  Constant8/1 -> Sum1/2
  Sum6/1 -> 1/2, Slope/1
  Constant2/1 -> Sum6/1, Sum5/2
  Sum5/1 -> 1/1
  Constant3/1 -> Sum5/1
  Mux/1 -> concentric branch/1
  Mux1/1 -> excentric branch/1
  v_excentric <N/1 -> Mux1/2
  Mux2/1 -> excentric overshoot/1
  concentric branch/1 -> Sum9/1
  excentric branch/1 -> Sum2/1
  Constant5/1 -> Mux1/3, Mux2/1
  Sum1/1 -> Mux2/3

== system atrias_HW_boom_nmSt_kinSw_v4/Control/Behavior Control/Virtual Neuromuscular Control/Muscle Layer/BFSH/PE force-length relation ==
  note: Parallel Elasticity PE
  lce [lopt] : Inport
  Constant3 : Constant
  Math Function2 : Math  Operator=square  SaturateOnIntegerOverflow=on
  Mux : Mux  Inputs=2
  Sum1 : Sum  Inputs=|+-  SaturateOnIntegerOverflow=on  InputSameDT=on  OutDataTypeStr=Inherit: Same as first input
  force above slack length : Fcn  Expr=u(2) * (u(1)>1)
  reference strain [lopt] : Constant  Value=mtu_w
  relative strain : Product  Inputs=*/
  fpe [Fmax] : Outport
  wires:
  Mux/1 -> force above slack length/1
  lce [lopt]/1 -> Mux/1, Sum1/1
  Constant3/1 -> Sum1/2
  Sum1/1 -> relative strain/1
  reference strain [lopt]/1 -> relative strain/2
  relative strain/1 -> Math Function2/1
  Math Function2/1 -> Mux/2
  force above slack length/1 -> fpe [Fmax]/1

== system atrias_HW_boom_nmSt_kinSw_v4/Control/Behavior Control/Virtual Neuromuscular Control/Muscle Layer/BFSH/SE force-length relation ==
  note: SE Force-Length Relationship
  lse [lslack] : Inport
  Constant1 : Constant
  Math Function : Math  Operator=square  SaturateOnIntegerOverflow=on
  Mux : Mux  Inputs=2
  Sum4 : Sum  Inputs=|+-  SaturateOnIntegerOverflow=on  InputSameDT=on  OutDataTypeStr=Inherit: Same as first input
  force above slack length : Fcn  Expr=u(2)*(u(1)>1)
  reference strain [lslack] : Constant  Value=mtu_eref
  relative strain : Product  Inputs=*/
  fse [Fmax] : Outport
  wires:
  Mux/1 -> force above slack length/1
  force above slack length/1 -> fse [Fmax]/1
  Math Function/1 -> Mux/2
  lse [lslack]/1 -> Mux/1, Sum4/1
  relative strain/1 -> Math Function/1
  reference strain [lslack]/1 -> relative strain/2
  Sum4/1 -> relative strain/1
  Constant1/1 -> Sum4/2

== system atrias_HW_boom_nmSt_kinSw_v4/Control/Behavior Control/Virtual Neuromuscular Control/Muscle Layer/BFSH1/BE force-length relation ==
  note: Buffer Elasticity BE
  lce [lopt] : Inport
  Constant1 : Constant  Value=1-mtu_w
  Math Function : Math  Operator=square  SaturateOnIntegerOverflow=on
  Mux1 : Mux  Inputs=2
  Sum4 : Sum  Inputs=|+-  SaturateOnIntegerOverflow=on  InputSameDT=on  OutDataTypeStr=Inherit: Same as first input
  force above slack length : Fcn  Expr=u(2)*(u(1)<0)
  reference strain [lslack] : Constant  Value=mtu_w/2
  relative strain : Product  Inputs=*/
  fbe [Fmax] : Outport
  wires:
  lce [lopt]/1 -> Sum4/1
  Mux1/1 -> force above slack length/1
  force above slack length/1 -> fbe [Fmax]/1
  Math Function/1 -> Mux1/2
  relative strain/1 -> Math Function/1
  reference strain [lslack]/1 -> relative strain/2
  Sum4/1 -> relative strain/1, Mux1/1
  Constant1/1 -> Sum4/2

== system atrias_HW_boom_nmSt_kinSw_v4/Control/Behavior Control/Virtual Neuromuscular Control/Muscle Layer/BFSH1/CE force-length relation ==
  note: CE Force-Length Relationship
  lce [lopt] : Inport
  Abs : Abs
  Constant1 : Constant
  Constant2 : Constant  Value=3
  Gain : Gain  Gain=log(mtu_c)
  Math Function : Math  SaturateOnIntegerOverflow=on
  Math Function1 : Math  Operator=pow  SaturateOnIntegerOverflow=on
  Sum4 : Sum  Inputs=|+-  SaturateOnIntegerOverflow=on  InputSameDT=on  OutDataTypeStr=Inherit: Same as first input
  normalized position : Product  Inputs=*/
  relative width : Constant  Value=mtu_w
  fce [Fmax] : Outport
  wires:
  lce [lopt]/1 -> Sum4/1
  relative width/1 -> normalized position/2
  Constant1/1 -> Sum4/2
  Sum4/1 -> Abs/1
  Abs/1 -> normalized position/1
  normalized position/1 -> Math Function1/1
  Constant2/1 -> Math Function1/2
  Math Function1/1 -> Gain/1
  Gain/1 -> Math Function/1
  Math Function/1 -> fce [Fmax]/1

== system atrias_HW_boom_nmSt_kinSw_v4/Control/Behavior Control/Virtual Neuromuscular Control/Muscle Layer/BFSH1/CE inverse force-velocity relation ==
  note: CE Inverse Force-Velocity Relationship
  Fv[Fmax] : Inport
  1 : Product  Inputs=/*
  Constant{1,3..4,8} (4 alike) : Constant
  Constant2 : Constant  Value=mtu_N
  Constant5 : Constant  Value=mtu_N
  Curvature : Gain  Gain=mtu_K  SaturateOnIntegerOverflow=on  OutDataTypeStr=Inherit: Same as input  ParamDataTypeStr=Inherit: Same as input
  Curvature1 : Gain  Gain=7.56*mtu_K  SaturateOnIntegerOverflow=on  OutDataTypeStr=Inherit: Same as input  ParamDataTypeStr=Inherit: Same as input
  Mux : Mux  Inputs=2
  Mux1 : Mux  Inputs=3
  Mux2 : Mux  Inputs=3
  Slope : Gain  Gain=1e-2  SaturateOnIntegerOverflow=on  OutDataTypeStr=Inherit: Same as input  ParamDataTypeStr=Inherit: Same as input
  Sum1 : Sum  Inputs=|++  SaturateOnIntegerOverflow=on  InputSameDT=on  OutDataTypeStr=Inherit: Same as first input
  Sum2 : Sum  SaturateOnIntegerOverflow=on  InputSameDT=on  OutDataTypeStr=Inherit: Same as first input
  Sum3 : Sum  Inputs=++|  SaturateOnIntegerOverflow=on  InputSameDT=on  OutDataTypeStr=Inherit: Same as first input
  Sum4 : Sum  Inputs=|+-  SaturateOnIntegerOverflow=on  InputSameDT=on  OutDataTypeStr=Inherit: Same as first input
  Sum5 : Sum  Inputs=|-+  SaturateOnIntegerOverflow=on  InputSameDT=on  OutDataTypeStr=Inherit: Same as first input
  Sum6 : Sum  Inputs=-+|  SaturateOnIntegerOverflow=on  InputSameDT=on  OutDataTypeStr=Inherit: Same as first input
  Sum7 : Sum  Inputs=|++  SaturateOnIntegerOverflow=on  InputSameDT=on  OutDataTypeStr=Inherit: Same as first input
  Sum8 : Sum  Inputs=+-|  SaturateOnIntegerOverflow=on  InputSameDT=on  OutDataTypeStr=Inherit: Same as first input
  Sum9 : Sum  SaturateOnIntegerOverflow=on  InputSameDT=on  OutDataTypeStr=Inherit: Same as first input
  concentric branch : Fcn  Expr=u(1) * (u(2)<=1)
  excentric branch : Fcn  Expr=u(2) * (u(1)>1)*(u(1)<=u(3))
  excentric overshoot : Fcn  Expr=u(3) * (u(2)>u(1))
  v_concentric : Product  Inputs=*/
  v_excentric <N : Product  Inputs=*/
  v[vmax] : Outport
  wires:
  Curvature/1 -> Sum3/2
  Constant1/1 -> Sum4/2, Sum3/1
  Sum4/1 -> v_concentric/1
  Sum3/1 -> v_concentric/2
  1/1 -> Sum7/1, Curvature1/1
  Constant4/1 -> Sum7/2, Sum8/1
  Curvature1/1 -> Sum8/2
  Sum8/1 -> v_excentric <N/2
  Sum7/1 -> v_excentric <N/1
  v_concentric/1 -> Mux/1
  Fv[Fmax]/1 -> Sum4/1, Curvature/1, Sum6/2, Mux/2, Mux1/1, Mux2/2
  Sum9/1 -> v[vmax]/1
  Sum2/1 -> Sum9/2
  excentric overshoot/1 -> Sum2/2
  Slope/1 -> Sum1/1
  Constant8/1 -> Sum1/2
  Sum6/1 -> 1/2, Slope/1
  Constant2/1 -> Sum6/1, Sum5/2
  Sum5/1 -> 1/1
  Constant3/1 -> Sum5/1
  Mux/1 -> concentric branch/1
  Mux1/1 -> excentric branch/1
  v_excentric <N/1 -> Mux1/2
  Mux2/1 -> excentric overshoot/1
  concentric branch/1 -> Sum9/1
  excentric branch/1 -> Sum2/1
  Constant5/1 -> Mux1/3, Mux2/1
  Sum1/1 -> Mux2/3

== system atrias_HW_boom_nmSt_kinSw_v4/Control/Behavior Control/Virtual Neuromuscular Control/Muscle Layer/BFSH1/PE force-length relation ==
  note: Parallel Elasticity PE
  lce [lopt] : Inport
  Constant3 : Constant
  Math Function2 : Math  Operator=square  SaturateOnIntegerOverflow=on
  Mux : Mux  Inputs=2
  Sum1 : Sum  Inputs=|+-  SaturateOnIntegerOverflow=on  InputSameDT=on  OutDataTypeStr=Inherit: Same as first input
  force above slack length : Fcn  Expr=u(2) * (u(1)>1)
  reference strain [lopt] : Constant  Value=mtu_w
  relative strain : Product  Inputs=*/
  fpe [Fmax] : Outport
  wires:
  Mux/1 -> force above slack length/1
  lce [lopt]/1 -> Mux/1, Sum1/1
  Constant3/1 -> Sum1/2
  Sum1/1 -> relative strain/1
  reference strain [lopt]/1 -> relative strain/2
  relative strain/1 -> Math Function2/1
  Math Function2/1 -> Mux/2
  force above slack length/1 -> fpe [Fmax]/1

== system atrias_HW_boom_nmSt_kinSw_v4/Control/Behavior Control/Virtual Neuromuscular Control/Muscle Layer/BFSH1/SE force-length relation ==
  note: SE Force-Length Relationship
  lse [lslack] : Inport
  Constant1 : Constant
  Math Function : Math  Operator=square  SaturateOnIntegerOverflow=on
  Mux : Mux  Inputs=2
  Sum4 : Sum  Inputs=|+-  SaturateOnIntegerOverflow=on  InputSameDT=on  OutDataTypeStr=Inherit: Same as first input
  force above slack length : Fcn  Expr=u(2)*(u(1)>1)
  reference strain [lslack] : Constant  Value=mtu_eref
  relative strain : Product  Inputs=*/
  fse [Fmax] : Outport
  wires:
  Mux/1 -> force above slack length/1
  force above slack length/1 -> fse [Fmax]/1
  Math Function/1 -> Mux/2
  lse [lslack]/1 -> Mux/1, Sum4/1
  relative strain/1 -> Math Function/1
  reference strain [lslack]/1 -> relative strain/2
  Sum4/1 -> relative strain/1
  Constant1/1 -> Sum4/2

== system atrias_HW_boom_nmSt_kinSw_v4/Control/Behavior Control/Virtual Neuromuscular Control/Muscle Layer/GLU/BE force-length relation ==
  note: Buffer Elasticity BE
  lce [lopt] : Inport
  Constant1 : Constant  Value=1-mtu_w
  Math Function : Math  Operator=square  SaturateOnIntegerOverflow=on
  Mux1 : Mux  Inputs=2
  Sum4 : Sum  Inputs=|+-  SaturateOnIntegerOverflow=on  InputSameDT=on  OutDataTypeStr=Inherit: Same as first input
  force above slack length : Fcn  Expr=u(2)*(u(1)<0)
  reference strain [lslack] : Constant  Value=mtu_w/2
  relative strain : Product  Inputs=*/
  fbe [Fmax] : Outport
  wires:
  lce [lopt]/1 -> Sum4/1
  Mux1/1 -> force above slack length/1
  force above slack length/1 -> fbe [Fmax]/1
  Math Function/1 -> Mux1/2
  relative strain/1 -> Math Function/1
  reference strain [lslack]/1 -> relative strain/2
  Sum4/1 -> relative strain/1, Mux1/1
  Constant1/1 -> Sum4/2

== system atrias_HW_boom_nmSt_kinSw_v4/Control/Behavior Control/Virtual Neuromuscular Control/Muscle Layer/GLU/CE force-length relation ==
  note: CE Force-Length Relationship
  lce [lopt] : Inport
  Abs : Abs
  Constant1 : Constant
  Constant2 : Constant  Value=3
  Gain : Gain  Gain=log(mtu_c)
  Math Function : Math  SaturateOnIntegerOverflow=on
  Math Function1 : Math  Operator=pow  SaturateOnIntegerOverflow=on
  Sum4 : Sum  Inputs=|+-  SaturateOnIntegerOverflow=on  InputSameDT=on  OutDataTypeStr=Inherit: Same as first input
  normalized position : Product  Inputs=*/
  relative width : Constant  Value=mtu_w
  fce [Fmax] : Outport
  wires:
  lce [lopt]/1 -> Sum4/1
  relative width/1 -> normalized position/2
  Constant1/1 -> Sum4/2
  Sum4/1 -> Abs/1
  Abs/1 -> normalized position/1
  normalized position/1 -> Math Function1/1
  Constant2/1 -> Math Function1/2
  Math Function1/1 -> Gain/1
  Gain/1 -> Math Function/1
  Math Function/1 -> fce [Fmax]/1
